simulink model "HyperscaleDataCenter"  (R2025b)
settings: Solver=VariableStepAuto  StartTime=0.0  StopTime=10  FixedStep=5e-5  RelTol=1e-4
PostLoadFcn:
  | HyperscaleDataCenterParam
values from neighbouring files (symbols this model uses):
  baseVoltageDC = 800    [DataCenterBBUParam.m]    (also in HyperscaleDataCenterParam.m; UPSBESSParam.m)
  bess_Ki = bess.controller.Ki    [SSTBESSParam.m]
  bess_Kp = bess.controller.Kp    [SSTBESSParam.m]
  droopGain = 0.02    [HyperscaleDataCenterParam.m]    (also in SSTBESSParam.m; UPSBESSParam.m)
  peakShavingPowerLimit = 800e3    (= 800000)    [HyperscaleDataCenterParam.m]
  powerTau = 0.005    [HyperscaleDataCenterParam.m]
  Prated_batt = 40e3    (= 40000)    [HyperscaleDataCenterParam.m]
  tauPS = 0.1    [HyperscaleDataCenterParam.m]
  Ts = 50e-6    (= 5e-05)    [BBUParam.m]    (also in DataCenterBBUParam.m; HyperscaleDataCenterParam.m)
  Ts_PS = 1e-3    (= 0.001)    [HyperscaleDataCenterParam.m]
undefined symbols (not defined in the file or in its folder): bbu, DiscIntNeverNeededParam, dspblkCoreblockFVToolHelper, ee_sli_rtmsupport, gcbh, grid, rack, sst, ups
libraries: fl_lib x80, nesl_utility x42, datacenter_lib x20, ee_lib x17, simulink x10, eeGeneralControl x9, slpidlib x6, microgridRenewables_lib x4, eeTransforms x4, batteryecm_lib x3, eeSinusoidalMeasurementV2 x2, simulink_extras x1
(part 2 of 5)

== system HyperscaleDataCenter/Server Load/Racks ==
  Fault Flag : Step  Time=100  SampleTime=0
  Inference Load Profile : simulink/Sources/Repeating Sequence Stair  OutValues=[0.45 0.45 0.45 0.45 0.45 0.45 0.45 0.45 0.45 0.45 0.45 0.45 0.45 0.45 0.45 0.45 0.45 0.45 0.45 0.45 0.45 0.45 0.45 0.45 0.45 0.45 0.45 0.45 0.45 0.45 0.45 0.45 0.45 0.45 0.45 0.45 0.45 0.45 0.45 0.45 0.45 0.45 0.45 0.45 0.45 0.45 0.45 0.45 0.45 0.45 0.45 0.45 0.45 0.45 0.45 0.45 0.45 0.45 0.45 0.45 0.45 0.45 0.45 0.45 0.45 0.45 0.45 0.45 0.45 0.45 0.45 0.45 0.45 0.45 0.45 0.45 0.45 0.45 0.45 0.45 0.45 0.45 0.45 0.45 0.45 0.45 0.45 0.45 0.45 0.45 0.45 0.45 0.45 0.45 0.45 0.45 0.45 0.45 0.45 0.45 0.45 0.45 0.45 0.45 0.45 0.45 0.45 0.45 0.45 0.45 0.45 0.45 0.45 0.45 0.45 0.45 0.45 0.45 0.45 0.45 0.45 0.45 0.45 0.45 0.45 0.45 0.45 0.45 0.45 0.45 0.45 0.45 0.45 0.45 0.45 0.45 0.45 0.45 0.45 0.45 0.45 0.45 0.45 0.45 0.45 0.45 0.45 0.45 0.45 0.45 0.45 0.45 0.45 0.45 0.45 0.45 0.45 0.45 0.45 0.45 0.45 0.45 0.45 0.45 0.45 0.45 0.45 0.45 0.45 0.45 0.45 0.45 0.45 0.45 0.45 0.45 0.45 0.45 0.45 0.45 0.45 0.45 0.45 0.45 0.45 0.45 0.45 0.45 0.45 0.45 0.45 0.45 0.45 0.45 0.45 0.45 0.45 0.45 0.45 0.45 0.09792 0.8812 0.4279 0.4233 0.3951 0.4417 0.4922 0.06292 0.07732 0.07716 0.08177 0.1021 0.07545 0.07538 0.0924 0.07838 0.07719 0.07756 0.07213 0.06917 0.07997 0.07917 0.09005 0.08372 0.8883 0.395 0.4378 0.3804 0.4688 0.4112 0.435 0.4169 0.4791 0.4658 0.06822 0.08707 0.06749 0.09019 0.07126 0.0691 0.0677 0.07873 0.0822 0.06972 0.09072 0.08156 0.8746 0.8709 0.4262 0.4091 0.4048 0.4395 0.4748 0.4245 0.4055 0.4479 0.429 0.3665 0.4045 0.4714 0.4592 0.412 0.4376 0.4419 0.471 0.4189 0.07003 0.04838 0.895 0.8492 0.3764 0.3779 0.4436 0.4654 0.4773 0.4169 0.4407 0.4152 0.425 0.4544 0.3988 0.403 0.4129 0.4294 0.4127 0.4608 0.448 0.5082 0.488 0.07604 0.07374 0.8828 0.8487 0.8895 0.8686 0.4234 0.4136 0.4116 0.4926 0.4523 0.4112 0.4573 0.4259 0.4585 0.4447 0.4258 0.3953 0.4105 0.4388 0.4452 0.4246 0.4057 0.4629 0.461 0.4449 0.4118 0.4226 0.3916 0.4792 0.4054 0.4544 0.4422 0.4546 0.4636 0.4855 0.4428 0.4343 0.4361 0.4804 0.496 0.4654 0.08359 0.05836 0.9365 0.8733 0.8654 0.8816 0.3909 0.3729 0.4338 0.408 0.4353 0.4173 0.4143 0.4129 0.4105 0.4518 0.4138 0.4419 0.4321 0.4582 0.4547 0.4547 0.422 0.4017 0.4296 0.4526 0.3913 0.4435 0.4495 0.4317 0.4677 0.4235 0.4225 0.4667 0.4516 0.4693 0.4495 0.4467 0.4675 0.4545 0.4623 0.4515 0.06221 0.04899 0.9312 0.8749 0.8663 0.8873 0.926 0.905 0.9178 0.4357 0.4379 0.4777 0.3905 0.4219 0.397 0.4112 0.4424 0.5089 0.4003 0.4322 0.4532 0.4096 0.4489 0.42 0.4478 0.4644 0.4798 0.4303 0.4447 0.4595 0.4207 0.4654 0.3944 0.4434 0.4156 0.41 0.3876 0.4556 0.4292 0.4569 0.4059 0.4228 0.4467 0.471 0.4269 0.4556 0.4737 0.4611 0.4292 0.4135 0.5131 0.4519 0.5096 0.4613 0.4618 0.4503 0.4521 0.465 0.4763 0.4887 0.4663 0.452 0.4517 0.4822 0.4565 0.4513 0.07011 0.06193 0.8485 0.8057 0.8966 0.8706 0.8889 0.8317 0.9382 0.8992 0.8382 0.8641 0.9356 0.9258 0.8751 0.9035 0.3864 0.4364 0.4714 0.4297 0.4344 0.4233 0.4155 0.4023 0.4171 0.3797 0.4569 0.41 0.3875 0.4516 0.458 0.465 0.4682 0.4113 0.422 0.4504 0.4696 0.3887 0.4557 0.4087 0.4055 0.435 0.4462 0.4446 0.4058 0.4619 0.4235 0.4096 0.4491 0.4915 0.4487 0.459 0.4611 0.4459 0.4174 0.4369 0.4407 0.4201 0.4502 0.4439 0.3833 0.4343 0.4686 0.3734 0.4581 0.447 0.4466 0.4605 0.4764 0.4359 0.4648 0.4588 0.4284 0.482 0.4881 0.4619 0.4698 0.4712 0.468 0.4737 0.4825 0.4637 0.4685 0.4701 0.4169 0.5148 0.487 0.4029 0.08186 0.07302 0.9172 0.454 0.4338 0.4223 0.4524 0.0829 0.09584 0.08212 0.07362 0.0809 0.08177 0.08467 0.07087 0.08213 0.08117 0.1012 0.07572 0.08253 0.09758 0.06311 0.09566 0.8076 0.4108 0.4467 0.3881 0.4411 0.4352 0.4492 0.3972 0.5191 0.5043 0.09358 0.08902 0.06735 0.08693 0.07385 0.05875 0.07534 0.0795 0.08597 0.08079 0.07329 0.1075 0.0587 0.9195 0.8938 0.3881 0.3788 0.4343 0.4336 0.4024 0.4979 0.4252 0.4297 0.4954 0.4318 0.4639 0.4354 0.432 0.4799 0.4474 0.4941 0.4304 0.4456 0.05767 0.07131 0.9125 0.8774 0.4413 0.4065 0.4383 0.4395 0.4492 0.4592 0.4394 0.45 0.417 0.3811 0.5062 0.4515 0.4701 0.4504 0.4205 0.4655 0.4519 0.4443 0.07985 0.08406 0.8564 0.9054 0.8433 0.418 0.3852 0.3823 0.4163 0.4218 ...(+2623 chars)]  tsamp=0.01  OutMin=[]  OutMax=[]  OutDataTypeStr=double  OutputDataTypeScalingMode=double  OutDataType=fixdt(0,8)  ConRadixGroup=Best Precision: Vector-wise  OutScaling=2^-12
  Inference Rack : Subsystem
  PS Step : fl_lib/Physical Signals/Sources/PS Step  step_time=100 s  initial_value=1  final_value=0
  SPST Switch : ee_lib/Switches & Breakers/SPST Switch  R_closed=0.001 Ohm  G_open=1e-6 S  Threshold=0.5 V  Width=0 V  model_dynamics=0  t_on=1e-3 s  t_off=1e-3 s  initial_vT=0 V
      settings: InternalSimscapePortConfiguration="{\"Bottom\":[],\"Left\":[{\"id\":\"vT\",\"label\":\"vT\",\"type\":\"input\"},{\"id\":\"p\",\"label\":\"\",\"type\":\"foundation.electrical.electrical\"}],\"Right\":[{\"id\":\"n\",\"label\":\"\",\"type\":\"foundation.electrical.electrical\"}],\"Top\":[]}"
  Training Load Profile : simulink/Sources/Repeating Sequence Stair  OutValues=[0.45 0.45 0.45 0.45 0.45 0.45 0.45 0.45 0.45 0.45 0.45 0.45 0.45 0.45 0.45 0.45 0.45 0.45 0.45 0.45 0.45 0.45 0.45 0.45 0.45 0.45 0.45 0.45 0.45 0.45 0.45 0.45 0.45 0.45 0.45 0.45 0.45 0.45 0.45 0.45 0.45 0.45 0.45 0.45 0.45 0.45 0.45 0.45 0.45 0.45 0.45 0.45 0.45 0.45 0.45 0.45 0.45 0.45 0.45 0.45 0.45 0.45 0.45 0.45 0.45 0.45 0.45 0.45 0.45 0.45 0.45 0.45 0.45 0.45 0.45 0.45 0.45 0.45 0.45 0.45 0.45 0.45 0.45 0.45 0.45 0.45 0.45 0.45 0.45 0.45 0.45 0.45 0.45 0.45 0.45 0.45 0.45 0.45 0.45 0.45 0.45 0.45 0.45 0.45 0.45 0.45 0.45 0.45 0.45 0.45 0.45 0.45 0.45 0.45 0.45 0.45 0.45 0.45 0.45 0.45 0.45 0.45 0.45 0.45 0.45 0.45 0.45 0.45 0.45 0.45 0.45 0.45 0.45 0.45 0.45 0.45 0.45 0.45 0.45 0.45 0.45 0.45 0.45 0.45 0.45 0.45 0.45 0.45 0.45 0.45 0.45 0.45 0.45 0.45 0.45 0.45 0.45 0.45 0.45 0.45 0.45 0.45 0.45 0.45 0.45 0.45 0.45 0.45 0.45 0.45 0.45 0.45 0.45 0.45 0.45 0.45 0.45 0.45 0.45 0.45 0.45 0.45 0.45 0.45 0.45 0.45 0.45 0.45 0.45 0.45 0.45 0.45 0.45 0.45 0.45 0.45 0.45 0.45 0.45 0.45 0.04462 0.05867 0.05976 0.05337 0.8301 0.8395 0.8241 0.8683 0.8535 0.8651 0.8382 0.8869 0.8863 0.8475 0.8278 0.8364 0.8503 0.8488 0.8368 0.8561 0.8418 0.8244 0.8443 0.8487 0.87 0.834 0.8518 0.8555 0.8073 0.8581 0.8308 0.8435 0.8996 0.8808 0.9365 0.9168 0.9028 0.928 0.9155 0.8937 0.9196 0.9024 0.9422 0.9107 0.9333 0.9094 0.9208 0.9231 0.9136 0.9629 0.936 0.9439 0.962 0.9278 0.9409 0.8926 0.9008 0.8666 0.9039 0.911 0.9053 0.9423 0.9029 0.9048 0.922 0.903 0.9312 0.9131 0.9474 0.9348 0.1393 0.1621 0.1647 0.1641 0.1161 0.1423 0.1202 0.1752 0.1554 0.1462 0.03853 0.04299 0.04355 0.05782 0.8563 0.8755 0.8485 0.8039 0.8697 0.8705 0.8526 0.862 0.8499 0.8518 0.8477 0.8228 0.8343 0.8033 0.8582 0.8377 0.8507 0.8641 0.8327 0.8442 0.8603 0.82 0.8209 0.834 0.8171 0.8803 0.8646 0.8542 0.8717 0.8626 0.9025 0.9584 0.9219 0.9301 0.9405 0.9014 0.9022 0.9003 0.9194 0.9374 0.9017 0.9207 0.915 0.8988 0.9028 0.9129 0.9366 0.9126 0.9212 0.9312 0.9165 0.941 0.9403 0.901 0.9198 0.913 0.8863 0.899 0.9338 0.9201 0.9109 0.9087 0.9491 0.9004 0.8974 0.9194 0.1738 0.1368 0.1536 0.1603 0.1415 0.1648 0.1441 0.1628 0.1555 0.1524 0.03233 0.05598 0.04442 0.03802 0.8071 0.8545 0.8574 0.8124 0.8511 0.836 0.8543 0.8144 0.8604 0.8429 0.8897 0.823 0.8373 0.8342 0.8774 0.8788 0.8398 0.856 0.8909 0.8535 0.8513 0.8096 0.8015 0.876 0.8889 0.8552 0.8426 0.8384 0.8708 0.8871 0.9413 0.9475 0.9331 0.875 0.8913 0.9496 0.9272 0.8941 0.8764 0.9402 0.897 0.9037 0.923 0.9311 0.9422 0.9095 0.9235 0.9039 0.9133 0.9329 0.9321 0.9474 0.9276 0.9244 0.8947 0.9106 0.9096 0.9026 0.9796 0.9135 0.9597 0.9275 0.9351 0.9202 0.9257 0.9193 0.1403 0.1602 0.139 0.1204 0.1525 0.1146 0.1697 0.1657 0.1804 0.1421 0.02264 0.06067 0.04766 0.06556 0.9084 0.8597 0.8401 0.8455 0.8659 0.8389 0.8325 0.8531 0.8901 0.871 0.8519 0.8336 0.8585 0.8754 0.834 0.8509 0.8686 0.8723 0.8567 0.8657 0.8408 0.8402 0.8673 0.8638 0.8755 0.8616 0.8501 0.8501 0.8618 0.854 0.931 0.9269 0.9581 0.9168 0.9116 0.8967 0.9258 0.8969 0.9188 0.9255 0.9006 0.9285 0.8993 0.9102 0.9354 0.911 0.9015 0.922 0.9323 0.8861 0.9272 0.8821 0.9023 0.9217 0.9231 0.9247 0.9276 0.9776 0.9213 0.9161 0.9361 0.907 0.9151 0.9014 0.9016 0.933 0.1643 0.1611 0.1483 0.1246 0.1351 0.1419 0.1511 0.1562 0.163 0.1382 0.06428 0.05871 0.05155 0.05442 0.8481 0.8333 0.8448 0.8584 0.8254 0.8387 0.8364 0.8278 0.8948 0.8577 0.8496 0.8168 0.8493 0.8486 0.8307 0.8452 0.8476 0.8629 0.8632 0.8297 0.8481 0.8635 0.8502 0.873 0.862 0.8265 0.8026 0.8657 0.8049 0.8561 0.9582 0.9256 0.9125 0.9248 0.9163 0.9241 0.9512 0.9099 0.9535 0.9364 0.906 0.9023 0.8988 0.9098 0.9292 0.8887 0.9103 0.9459 0.8959 0.9341 0.9067 0.8909 0.9301 0.934 0.9283 0.9331 0.9562 0.9058 0.9018 0.9366 0.9405 0.959 0.9171 0.9144 0.9386 0.9049 0.04418 0.03775 0.02733 0.04007 0.03547 0.01946 0.04286 0.03016 0.0388 0.02572 0.05602 0.04867 0.02169 0.06863 0.829 0.8294 0.8837 0.8772 0.8545 0.8538 0.8485 0.8357 0.8388 0.8571 0.8782 0.8747 0.8593 0.8062 0.8493 0.7853 0.8512 0.8453 0.8751 0.8385 0.8044 0.8229 0.8738 0.8612 0.8137 ...(+2573 chars)]  tsamp=0.01  OutMin=[]  OutMax=[]  OutDataTypeStr=double  OutputDataTypeScalingMode=double  OutDataType=fixdt(0,8)  ConRadixGroup=Best Precision: Vector-wise  OutScaling=2^-12
  Training Rack : Subsystem
  + : PMIOPort  Side=Left
  - : PMIOPort  Port=2  Side=Left
  wires:
  Training Load Profile/1 -> Training Rack/1(U_in)
  Inference Load Profile/1 -> Inference Rack/1(U_in)
  Fault Flag/1 -> Inference Rack/2(FaultFlag), Training Rack/2(FaultFlag)
  connections:
  SPST Switch/RConn1 -- Training Rack/LConn1
  PS Step/RConn1 -- SPST Switch/LConn1
  +/RConn1 -- SPST Switch/LConn2 -- Inference Rack/LConn1
  Training Rack/LConn2 -- -/RConn1 -- Inference Rack/LConn2

== system HyperscaleDataCenter/Solid State Transformer/Converters ==
  note: DAB Phase shift signal
  note: Reference signal for H-Bridge
  mabc : Inport
  phi : Inport  Port=2
  Add : Sum  Inputs=+++
  Add1 : Sum  Inputs=+++
  Bus Creator : BusCreator  Inputs=5
  Demux : Demux  Outputs=3
  Demux1 : Demux  Outputs=3
  Electrical Reference1 : fl_lib/Electrical/Electrical Elements/Electrical Reference
  Gain_1_1 : Gain  Gain=1/3
  Gain_1_3 : Gain  Gain=1/3
  Phase Splitter : ee_lib/Connectors & References/Phase Splitter
  Subsystem1 : Subsystem
  Subsystem2 : Subsystem
  Subsystem3 : Subsystem
  ABC2 : PMIOPort  Side=Left
  + : PMIOPort  Port=2  Side=Right
  - : PMIOPort  Port=3  Side=Right
  Vdc : Outport
  VdcMeas : Outport  Port=2
  wires:
  Subsystem1/1(Out1) -> Bus Creator/1, Add/1  "AVdc"
  Subsystem2/1(Out1) -> Add/2, Bus Creator/2  "BAVdc"
  Subsystem3/1(Out1) -> Bus Creator/3, Add/3  "CVdc"
  Add/1 -> Gain_1_3/1
  Gain_1_3/1 -> VdcMeas/1, Bus Creator/4  "AvGVdc"
  Bus Creator/1 -> Vdc/1
  phi/1 -> Demux1/1
  Subsystem2/2(V_out_pu) -> Add1/2
  Subsystem1/2(V_out_pu) -> Add1/1
  Subsystem3/2(V_out_pu) -> Add1/3
  Add1/1 -> Gain_1_1/1
  Gain_1_1/1 -> Bus Creator/5  "PUVdc"
  Demux1/1 -> Subsystem1/1(PhA)
  Demux1/2 -> Subsystem2/1(PhB)
  Demux1/3 -> Subsystem3/1(PhC)
  mabc/1 -> Demux/1
  Demux/1 -> Subsystem1/2(ma)
  Demux/2 -> Subsystem2/2(mb)
  Demux/3 -> Subsystem3/2(mc)
  connections:
  Subsystem1/LConn2 -- Subsystem2/LConn2 -- Subsystem3/LConn2 -- Electrical Reference1/LConn1
  Subsystem3/LConn1 -- Phase Splitter/RConn3
  Subsystem1/LConn1 -- Phase Splitter/RConn1
  Subsystem1/RConn2 -- Subsystem3/RConn2 -- -/RConn1 -- Subsystem2/RConn2
  Subsystem2/LConn1 -- Phase Splitter/RConn2
  Subsystem1/RConn1 -- Subsystem3/RConn1 -- Subsystem2/RConn1 -- +/RConn1
  Phase Splitter/LConn1 -- ABC2/RConn1

== system HyperscaleDataCenter/Solid State Transformer/DAB Controller ==
  Vdc : Inport
  Vac : Inport  Port=2
  AND_gate : Logic  AllPortsSameDT=off  OutDataTypeStr=boolean
  AND_reset : Logic  AllPortsSameDT=off  OutDataTypeStr=boolean
  Add : Sum
  Add1 : Sum
  Add2 : Sum
  Bus Selector : BusSelector  OutputSignals=AVdc,BAVdc,CVdc,AvGVdc,PUVdc
  Bus Selector1 : BusSelector  OutputSignals=pllVmag [pu],reset
  Constant : Constant  Value=0
  DAB Balancing : Subsystem
  Error : Sum  Inputs=+-
  Mux : Mux  Inputs=3
  Mux1 : Mux  Inputs=3
  PI_central : slpidlib/PID Controller  Controller=PI  Form=Parallel  TimeDomain=Discrete-time  UseExternalTs=off  SampleTime=sst.dab.sampleTime  IntegratorMethod=Forward Euler  FilterMethod=Forward Euler  ControllerParametersSource=internal  P=sst.dab.kp  I=sst.dab.ki  UseKiTs=off  D=0  UseExternalDerivativeSource=off  N=100  UseFilter=on  TunerSelectOption=Transfer Function Based (PID Tuner App)  InitialConditionSource=internal  InitialConditionForIntegrator=0  InitialConditionForFilter=0  DifferentiatorICPrevScaledInput=0  ExternalReset=falling  TrackingMode=off  Kt=1  LimitOutput=on  SatLimitsSource=internal  UpperSaturationLimit=sst.dab.upperLimit  LowerSaturationLimit=sst.dab.lowerLimit  LinearizeAsGain=off  AntiWindupMode=none  Kb=1  LimitIntegrator=off  UpperIntegratorSaturationLimit=inf  LowerIntegratorSaturationLimit=-inf  POutMin=[]  POutMax=[]  IOutMin=[]  IOutMax=[]  DOutMin=[]  DOutMax=[]  NOutMin=[]  NOutMax=[]  SumOutMin=[]  SumOutMax=[]  SaturationOutMin=[]  SaturationOutMax=[]  PParamMin=[]  PParamMax=[]  IParamMin=[]  IParamMax=[]  DParamMin=[]  DParamMax=[]  NParamMin=[]  NParamMax=[]  KbParamMin=[]  KbParamMax=[]  KtParamMin=[]  KtParamMax=[]  KbOutMin=[]  KbOutMax=[]  KtOutMin=[]  KtOutMax=[]  IntegratorOutMin=[]  IntegratorOutMax=[]  FilterOutMin=[]  FilterOutMax=[]  SumI1OutMin=[]  SumI1OutMax=[]  SumI2OutMin=[]  SumI2OutMax=[]  SumI3OutMin=[]  SumI3OutMax=[]  SumI4OutMin=[]  SumI4OutMax=[]  SumDOutMin=[]  SumDOutMax=[]  DifferentiatorOutMin=[]  DifferentiatorOutMax=[]  FilterDiffOutCoefMin=[]  FilterDiffOutCoefMax=[]  ReciprocalOutMin=[]  ReciprocalOutMax=[]  SumDenOutMin=[]  SumDenOutMax=[]  SumNumOutMin=[]  SumNumOutMax=[]  DivideOutMin=[]  DivideOutMax=[]  UdiffTsProdOutMin=[]  UdiffTsProdOutMax=[]  NTsProdOutMin=[]  NTsProdOutMax=[]  UintegralTsProdOutMin=[]  UintegralTsProdOutMax=[]  UngainTsProdOutMin=[]  UngainTsProdOutMax=[]  ClampingZeroOutDataTypeStr=Inherit: Inherit via back propagation  ClampingZeroOutMin=[]  ClampingZeroOutMax=[]  FilterDenConstantOutDataTypeStr=Inherit: Inherit via back propagation  FilterDenConstantOutMin=[]  FilterDenConstantOutMax=[]  PCopyOutDataTypeStr=Inherit: Inherit via back propagation  PCopyOutMin=[]  PCopyOutMax=[]  NCopyOutDataTypeStr=Inherit: Inherit via back propagation  NCopyOutMin=[]  NCopyOutMax=[]  IntegratorContinuousStateAttributes=''  IntegratorStateMustResolveToSignalObject=off  IntegratorRTWStateStorageClass=Auto  FilterContinuousStateAttributes=''  FilterStateMustResolveToSignalObject=off  FilterRTWStateStorageClass=Auto  ParallelPVariant=InternalParameters  IdealPVariant=Disabled  IVariant=InternalParameters  DVariant=Disabled  IntegratorVariant=Discrete  SatVariant=Enabled  AWVariant=Passthrough  PCopyVariant=Disabled  TRVariant=Disabled  FdbkBlocksVariant=Forward  IdealPFdbkVariant=Disabled  SatFdbkVariant=Disabled  DerivativeFilterVariant=Disabled  NVariant=Disabled  NCopyVariant=Disabled_SignalSpec  FilterICVariant=Disabled  IntegratorICVariant=InternalICs  ExternalResetVariant=ExternalReset  TRSumVariant=Passthrough  SumFdbkVariant=Disabled  SumVariant=Sum_PI  TsampFilterVariant=InternalTs  TsampNgainVariant=Passthrough  TsampIntegralVariant=Disabled_SignalSpec  ExternalSaturationOutDataTypeStr=Inherit: Same as second input  DerivativeSourceVariant=Disabled  PreIntVariant=InternalPreInt
      settings: LibrarySourceBlock=simulink/Discrete/Discrete PID Controller
  StartupDelay : Step  SampleTime=0
  Switch : Switch  Criteria=u2 > Threshold  SaturateOnIntegerOverflow=off  InputSameDT=off
  VacLowRelay : Relay  OnSwitchValue=0.48  OffSwitchValue=0.42  OnOutputValue=0  OffOutputValue=1
  Vref : Constant
  phi : Outport
  wires:
  Vref/1 -> Error/1
  Error/1 -> PI_central/1
  PI_central/1 -> Add1/1, Add2/1, Add/1
  Vdc/1 -> Bus Selector/1
  Bus Selector/1 -> DAB Balancing/1(Vdc_A)  "<AVdc>"
  Bus Selector/2 -> DAB Balancing/2(Vdc_B)  "<BAVdc>"
  Bus Selector/3 -> DAB Balancing/3(Vdc_C)  "<CVdc>"
  Bus Selector/4 -> DAB Balancing/4(Vdc_avg)  "<AvGVdc>"
  Bus Selector/5 -> Error/2  "<PUVdc>"
  DAB Balancing/1(delta_d_A) -> Add/2  "delta_d_A"
  DAB Balancing/2(delta_d_B) -> Add1/2  "delta_d_B"
  DAB Balancing/3(delta_d_C) -> Add2/2  "delta_d_C"
  Add/1 -> Mux/1
  Add2/1 -> Mux/3
  Add1/1 -> Mux/2
  Mux/1 -> Switch/3
  Vac/1 -> Bus Selector1/1
  Bus Selector1/1 -> VacLowRelay/1  "<pllVmag [pu]>"
  Switch/1 -> phi/1
  Constant/1 -> Mux1/3, Mux1/2, Mux1/1
  Mux1/1 -> Switch/1
  StartupDelay/1 -> AND_gate/2, AND_reset/2
  AND_gate/1 -> Switch/2
  Bus Selector1/2 -> AND_reset/1  "<reset>"
  AND_reset/1 -> PI_central/2
  VacLowRelay/1 -> AND_gate/1

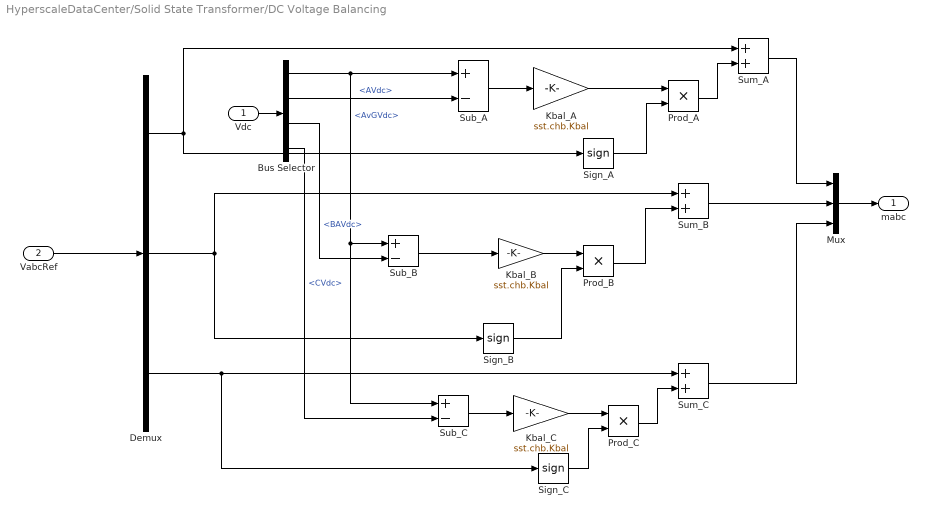
== system HyperscaleDataCenter/Solid State Transformer/DC Voltage Balancing ==
  Vdc : Inport
  VabcRef : Inport  Port=2
  Bus Selector : BusSelector  OutputSignals=AvGVdc,AVdc,BAVdc,CVdc
  Demux : Demux  Outputs=3
  Kbal_A : Gain  Gain=sst.chb.Kbal
  Kbal_B : Gain  Gain=sst.chb.Kbal
  Kbal_C : Gain  Gain=sst.chb.Kbal
  Mux : Mux  Inputs=3
  Prod_A : Product
  Prod_B : Product
  Prod_C : Product
  Sign_A : Signum
  Sign_B : Signum
  Sign_C : Signum
  Sub_A : Sum  Inputs=+-
  Sub_B : Sum  Inputs=+-
  Sub_C : Sum  Inputs=+-
  Sum_A : Sum
  Sum_B : Sum
  Sum_C : Sum
  mabc : Outport
  wires:
  Sub_B/1 -> Kbal_B/1
  Prod_B/1 -> Sum_B/2
  Sub_A/1 -> Kbal_A/1
  Sub_C/1 -> Kbal_C/1
  Kbal_A/1 -> Prod_A/1
  Sign_A/1 -> Prod_A/2
  Kbal_C/1 -> Prod_C/1
  Sign_C/1 -> Prod_C/2
  Kbal_B/1 -> Prod_B/1
  Sign_B/1 -> Prod_B/2
  Prod_A/1 -> Sum_A/2
  Prod_C/1 -> Sum_C/2
  Bus Selector/1 -> Sub_C/1, Sub_B/1, Sub_A/1  "<AvGVdc>"
  VabcRef/1 -> Demux/1
  Demux/1 -> Sum_A/1, Sign_A/1
  Demux/2 -> Sum_B/1, Sign_B/1
  Demux/3 -> Sign_C/1, Sum_C/1
  Sum_B/1 -> Mux/2
  Sum_A/1 -> Mux/1
  Sum_C/1 -> Mux/3
  Mux/1 -> mabc/1
  Vdc/1 -> Bus Selector/1
  Bus Selector/2 -> Sub_A/2  "<AVdc>"
  Bus Selector/3 -> Sub_B/2  "<BAVdc>"
  Bus Selector/4 -> Sub_C/2  "<CVdc>"

== system HyperscaleDataCenter/Solid State Transformer/Filter & AC measurements ==
  Current : Subsystem
  Current and Voltage Sensor (Three-Phase) : ee_lib/Sensors & Transducers/Current and Voltage Sensor (Three-Phase)  vMeasurementType=ee.enum.vmeasurement.lg  outputUnit=ee.enum.unit.pu  SRated=20e6 A*V  VRated=13800 V  I_specify=off  I_priority=None  I=[0, 0, 0] A  I_nominal_specify=off  I_nominal_value=1  I_nominal_unit=A  V_specify=off  V_priority=None  V=[0, 0, 0] V  V_nominal_specify=off  V_nominal_value=1  V_nominal_unit=V
      settings: InternalSimscapePortConfiguration="{\"Bottom\":[],\"Left\":[{\"id\":\"N1\",\"label\":\"~1\",\"type\":\"foundation.electrical.three_phase\"}],\"Right\":[{\"id\":\"V_output\",\"label\":\"V\",\"type\":\"output\"},{\"id\":\"I_output\",\"label\":\"I\",\"type\":\"output\"},{\"id\":\"N2\",\"label\":\"~2\",\"type\":\"foundation.electrical.three_phase\"}],\"Top\":[]}"
  Gain : Gain  Gain=1/(5e6)
  Gain1 : Gain  Gain=1/(5e6)
  Low-Pass Filter (Discrete or Continuous)1 : eeGeneralControl/Low-Pass Filter (Discrete or Continuous)  K=1  T=10e-3  B=inf  A=-inf  init_option=Inherited from block input  x0=0  Ts=-1
  Low-Pass Filter (Discrete or Continuous)2 : eeGeneralControl/Low-Pass Filter (Discrete or Continuous)  K=1  T=10e-3  B=inf  A=-inf  init_option=Inherited from block input  x0=0  Ts=-1
  PLL : Subsystem  Commented=on
      settings: PortSchema="{\"entries\":[{\"content\":{\"sides\":[{\"content\":{\"connectorIds\":[\"Out1\",\"Out2\",\"Out3\"]},\"type\":\"ConnectorPlacement.EquallySpacedRectSide\",\"uuid\":\"76485780-20fe-4fcf-8224-69648da6ed2a\"},{\"content\":{\"connectorIds\":[\"In1\",\"In2\"],\"side\":\"RIGHT\"},\"type\":\"ConnectorPlacement.EquallySpacedRectSide\",\"uuid\":\"f19a6390-e634-42c7-8d46-4cd80cbab182\"},{\"content\":{\"side\":\"TOP\"},\"type\":\"ConnectorPlacement.EquallySpacedRectSide\",\"uuid\":\"87682f72-1844-428e-be70-ad7ca3191ee3\"}]},\"type\":\"ConnectorPlacement.EquallySpacedConnector\",\"uuid\":\"f2136b07-48ec-402b-adb3-18c0bac2157c\"}],\"packageUris\":[\"http://schema.mathworks.com/mf0/Connector/R2020b\"],\"version\":\"1.0\"}"
  PS-Simulink Converter : nesl_utility/PS-Simulink Converter  PhysicalDomain=network_engine_domain  SubClassName=ps_output  LeftPortType=input  RightPortType=output  PseudoPeriodic=off  Frequencies=[]  VectorFormat=1-D array  Unit=inherit  AffineConversion=off
  PS-Simulink Converter1 : nesl_utility/PS-Simulink Converter  PhysicalDomain=network_engine_domain  SubClassName=ps_output  LeftPortType=input  RightPortType=output  PseudoPeriodic=off  Frequencies=[]  VectorFormat=1-D array  Unit=inherit  AffineConversion=off
  PS-Simulink Converter2 : nesl_utility/PS-Simulink Converter  PhysicalDomain=network_engine_domain  SubClassName=ps_output  LeftPortType=input  RightPortType=output  PseudoPeriodic=off  Frequencies=[]  VectorFormat=inherit  Unit=inherit  AffineConversion=off
  PS-Simulink Converter3 : nesl_utility/PS-Simulink Converter  PhysicalDomain=network_engine_domain  SubClassName=ps_output  LeftPortType=input  RightPortType=output  PseudoPeriodic=off  Frequencies=[]  VectorFormat=inherit  Unit=inherit  AffineConversion=off
  Power Sensor (Three-Phase) : ee_lib/Sensors & Transducers/Power Sensor (Three-Phase)  load_type=ee.enum.passive.type_balanced.balanced  f0=60 Hz
      settings: InternalSimscapePortConfiguration="{\"Bottom\":[],\"Left\":[{\"id\":\"N1\",\"label\":\"~1\",\"type\":\"foundation.electrical.three_phase\"}],\"Right\":[{\"id\":\"N2\",\"label\":\"~2\",\"type\":\"foundation.electrical.three_phase\"}],\"Top\":[{\"id\":\"Pm\",\"label\":\"P\",\"type\":\"output\"},{\"id\":\"Qm\",\"label\":\"Q\",\"type\":\"output\"}]}"
  RL filter : ee_lib/Passive/RLC Assemblies/RLC (Three-Phase)  port_option=ee.enum.threePhasePort.composite  component_structure=ee.enum.rlc.structure.SeriesRL  R=0.1 Ohm  L=0.01 H  C=1e-6 F  R_parasitic=1e-6 Ohm  G_parasitic=1e-6 1/Ohm  IL_specify=on  IL_priority=None  IL=[0, 0, 0] A  IL_nominal_specify=off  IL_nominal_value=1  IL_nominal_unit=A  VC_specify=on  VC_priority=None  VC=[0, 0, 0] V  VC_nominal_specify=off  VC_nominal_value=1  VC_nominal_unit=V
      settings: InternalSimscapePortConfiguration="{\"Bottom\":[],\"Left\":[{\"id\":\"N1\",\"label\":\"~1\",\"type\":\"foundation.electrical.three_phase\"}],\"Right\":[{\"id\":\"N2\",\"label\":\"~2\",\"type\":\"foundation.electrical.three_phase\"}],\"Top\":[]}"
  Terminator : Terminator
  Terminator1 : Terminator
  Voltage : Subsystem
  ABC : PMIOPort  Side=Left
  ABC2 : PMIOPort  Port=2  Side=Right
  Vabc : Outport
  Iabc : Outport  Port=2
  wires:
  PS-Simulink Converter/1 -> Current/1(Isabc)
  Current/1(Iabc) -> Iabc/1, PLL/1(Iabc)
  PS-Simulink Converter1/1 -> Voltage/1(Vsabc)
  Voltage/1(Vabc) -> Vabc/1, PLL/2(V)
  PS-Simulink Converter2/1 -> Gain/1
  PS-Simulink Converter3/1 -> Gain1/1
  Gain/1 -> Low-Pass Filter (Discrete or Continuous)1/1
  Gain1/1 -> Low-Pass Filter (Discrete or Continuous)2/1
  PLL/3(mag) -> ?
  PLL/2(freq) -> ?
  Low-Pass Filter (Discrete or Continuous)1/1 -> Terminator/1
  Low-Pass Filter (Discrete or Continuous)2/1 -> Terminator1/1
  connections:
  Current and Voltage Sensor (Three-Phase)/RConn2 -- PS-Simulink Converter/LConn1
  PS-Simulink Converter1/LConn1 -- Current and Voltage Sensor (Three-Phase)/RConn1
  Current and Voltage Sensor (Three-Phase)/LConn1 -- ABC/RConn1
  Power Sensor (Three-Phase)/RConn1 -- RL filter/LConn1
  Power Sensor (Three-Phase)/LConn2 -- PS-Simulink Converter2/LConn1
  Power Sensor (Three-Phase)/LConn3 -- PS-Simulink Converter3/LConn1
  RL filter/RConn1 -- ABC2/RConn1
  Power Sensor (Three-Phase)/LConn1 -- Current and Voltage Sensor (Three-Phase)/RConn3

== system HyperscaleDataCenter/Solid State Transformer/PFC Rectifier Controller ==
  VdcRef (V) : Inport
  QRef (pu) : Inport  Port=2
  VdcSens (V) : Inport  Port=3
  VabcSens (pu) : Inport  Port=4
  IabcSens (pu) : Inport  Port=5
  Current Controller : Subsystem
  DC Voltage Controller and Current Reference : Subsystem
  PLL : Subsystem
      settings: PortSchema="{\"entries\":[{\"content\":{\"sides\":[{\"content\":{\"connectorIds\":[\"Out1\",\"Out2\",\"Out3\",\"Out4\"]},\"type\":\"ConnectorPlacement.EquallySpacedRectSide\",\"uuid\":\"76485780-20fe-4fcf-8224-69648da6ed2a\"},{\"content\":{\"connectorIds\":[\"In1\"],\"side\":\"RIGHT\"},\"type\":\"ConnectorPlacement.EquallySpacedRectSide\",\"uuid\":\"f19a6390-e634-42c7-8d46-4cd80cbab182\"},{\"content\":{\"side\":\"TOP\"},\"type\":\"ConnectorPlacement.EquallySpacedRectSide\",\"uuid\":\"87682f72-1844-428e-be70-ad7ca3191ee3\"}]},\"type\":\"ConnectorPlacement.EquallySpacedConnector\",\"uuid\":\"f2136b07-48ec-402b-adb3-18c0bac2157c\"}],\"packageUris\":[\"http://schema.mathworks.com/mf0/Connector/R2020b\"],\"version\":\"1.0\"}"
  Rate Transition : RateTransition  InitialCondition=1  OutPortSampleTime=Ts
  Reset Controller : Subsystem
  VabcRef (pu) : Outport
  Out Bus Element : Outport  Port=2  PortName=Visualization  Element=pllAngle [rad]
  Out Bus Element1 : Outport  Port=2  PortName=Visualization  Element=pllVmag [pu]
  Out Bus Element2 : Outport  Port=2  PortName=Visualization  Element=Idref [pu]
  Out Bus Element3 : Outport  Port=2  PortName=Visualization  Element=Iqref [pu]
  Out Bus Element5 : Outport  Port=2  PortName=Visualization  Element=IdCntrlError [pu]
  Out Bus Element6 : Outport  Port=2  PortName=Visualization  Element=IqCntrlError [pu]
  BusElementOut : Outport  Port=2  PortName=Visualization  Element=reset
  Flag : Outport  Port=3
  wires:
  Current Controller/3(IqCntrlError) -> Out Bus Element6/1
  Current Controller/2(IdCntrlError) -> Out Bus Element5/1
  PLL/1(theta) -> Out Bus Element/1, Current Controller/3(theta)
  Rate Transition/1 -> PLL/1(V)
  DC Voltage Controller and Current Reference/2(iqRef) -> Current Controller/2(iqRef), Out Bus Element3/1
  DC Voltage Controller and Current Reference/1(idRef) -> Out Bus Element2/1, Current Controller/1(idRef)
  IabcSens (pu)/1 -> Current Controller/6(iabc(PU))
  PLL/3(Vq) -> Current Controller/5(vq)
  VdcSens (V)/1 -> DC Voltage Controller and Current Reference/4(VdcSens)
  Current Controller/1(vabcRef) -> VabcRef (pu)/1
  PLL/4(mag) -> Current Controller/7(Vmag), Reset Controller/1(u), DC Voltage Controller and Current Reference/2(vPeak), Out Bus Element1/1
  QRef (pu)/1 -> DC Voltage Controller and Current Reference/1(qRef)
  VabcSens (pu)/1 -> Rate Transition/1
  VdcRef (V)/1 -> DC Voltage Controller and Current Reference/3(vdcRef)
  PLL/2(Vd) -> Current Controller/4(vd)
  Current Controller/4(Flag) -> Flag/1
  Reset Controller/1(Out1) -> Current Controller/8(Reset), BusElementOut/1, DC Voltage Controller and Current Reference/5(Reset)

== system HyperscaleDataCenter/Battery Energy Storage/BESS/DC-DC Converter Controller ==
  Voref : Inport
  Vo : Inport  Port=2
  Vac : Inport  Port=3
  iPeakShave : Inport  Port=4
  Flag : Inport  Port=5
  Current Reference Generator : Subsystem
  Gain : Gain  Gain=18750
  Mode Control : Subsystem
  Saturation : Saturate  UpperLimit=0  LowerLimit=-40000
  Simulink-PS Converter : nesl_utility/Simulink-PS Converter  PhysicalDomain=network_engine_domain  SubClassName=ps_input  LeftPortType=input  RightPortType=output  PseudoPeriodic=off  Frequencies=[]  NoiseDistribution=none  NoiseParameters=[]  Unit=1  AffineConversion=off  FilteringAndDerivatives=filter  SimscapeFilterOrder=1  InputFilterTimeConstant=0.001  UdotUserProvided=0
  mod : PMIOPort  Side=Right
  wires:
  Gain/1 -> Saturation/1
  Vac/1 -> Mode Control/2(Vac)
  Current Reference Generator/1(i) -> Gain/1
  Mode Control/1(DischargeFlag) -> Current Reference Generator/2(DischargeFlag)
  Saturation/1 -> Simulink-PS Converter/1
  Vo/1 -> Mode Control/1(Vdc)
  Mode Control/3(iRef) -> Current Reference Generator/4(I)
  Voref/1 -> Current Reference Generator/1(VoRef)
  iPeakShave/1 -> Current Reference Generator/6(iPeakShave)
  Mode Control/2(vOut) -> Current Reference Generator/3(Vo)
  Flag/1 -> Current Reference Generator/5(Mode)
  connections:
  mod/RConn1 -- Simulink-PS Converter/RConn1

== system HyperscaleDataCenter/HV Substation/Transformer/Detailed ==
  Two-Winding Transformer (Three-Phase) : ee_lib/Passive/Transformers/Two-Winding Transformer (Three-Phase)  SRated=100e6 A*V  FRated=grid.frequency Hz  Winding1Connection=ee.enum.windingconnection.Yg  VRated1=grid.voltage V  Winding2Connection=ee.enum.windingconnection.Yg  VRated2=13800 V  CoreType=ee.enum.coretype.threelimb  pu_Rw1=0.01  pu_Rw2=0.01  leakage_reactance_option=ee.enum.transformer_leakage.include  pu_Xl1=0.05  pu_Xl2=0.05  magnetizing_resistance_option=ee.enum.transformer_magnetizingResistance.exclude  pu_Rm=500  magnetizing_reactance_option=ee.enum.transformer_magnetizingReactance.exclude  saturation_option=ee.enum.transformer_saturation.exclude  pu_Xm=500  current_data=[0, .002, 1, 2]  magnetic_flux_data=[0, 1.2, 1.5, 1.51]  pu_X0=0.5  i1_specify=off  i1_priority=None  i1=[0, 0, 0] A  i1_nominal_specify=off  i1_nominal_value=1  i1_nominal_unit=A  i2_specify=off  i2_priority=None  i2=[0, 0, 0] A  i2_nominal_specify=off  i2_nominal_value=1  i2_nominal_unit=A  phi_specify=off  phi_priority=None  phi=[0, 0, 0]  phi_nominal_specify=off  phi_nominal_value=1  phi_nominal_unit=1  power_dissipated_specify=off  power_dissipated_priority=None  power_dissipated=0 W  power_dissipated_nominal_specify=off  power_dissipated_nominal_value=1  power_dissipated_nominal_unit=W
      settings: InternalSimscapePortConfiguration="{\"Bottom\":[],\"Left\":[{\"id\":\"N1\",\"label\":\"~1\",\"type\":\"foundation.electrical.three_phase\"}],\"Right\":[{\"id\":\"N2\",\"label\":\"~2\",\"type\":\"foundation.electrical.three_phase\"}],\"Top\":[]}"
  In : PMIOPort  Side=Left
  Out : PMIOPort  Port=2  Side=Right
  connections:
  Two-Winding Transformer (Three-Phase)/LConn1 -- In/RConn1
  Two-Winding Transformer (Three-Phase)/RConn1 -- Out/RConn1

== system HyperscaleDataCenter/HV Substation/Transformer/Simplified ==
  Electrical Reference : fl_lib/Electrical/Electrical Elements/Electrical Reference
  Electrical Reference1 : fl_lib/Electrical/Electrical Elements/Electrical Reference
  Ideal Transformer : fl_lib/Electrical/Electrical Elements/Ideal Transformer  n=windingRatio  i1_specify=off  i1_priority=None  i1=0 A  i1_nominal_specify=off  i1_nominal_value=1  i1_nominal_unit=A  v1_specify=off  v1_priority=None  v1=0 V  v1_nominal_specify=off  v1_nominal_value=1  v1_nominal_unit=V  i2_specify=off  i2_priority=None  i2=0 A  i2_nominal_specify=off  i2_nominal_value=1  i2_nominal_unit=A  v2_specify=off  v2_priority=None  v2=0 V  v2_nominal_specify=off  v2_nominal_value=1  v2_nominal_unit=V
  Ideal Transformer1 : fl_lib/Electrical/Electrical Elements/Ideal Transformer  n=windingRatio  i1_specify=off  i1_priority=None  i1=0 A  i1_nominal_specify=off  i1_nominal_value=1  i1_nominal_unit=A  v1_specify=off  v1_priority=None  v1=0 V  v1_nominal_specify=off  v1_nominal_value=1  v1_nominal_unit=V  i2_specify=off  i2_priority=None  i2=0 A  i2_nominal_specify=off  i2_nominal_value=1  i2_nominal_unit=A  v2_specify=off  v2_priority=None  v2=0 V  v2_nominal_specify=off  v2_nominal_value=1  v2_nominal_unit=V
  Ideal Transformer2 : fl_lib/Electrical/Electrical Elements/Ideal Transformer  n=windingRatio  i1_specify=off  i1_priority=None  i1=0 A  i1_nominal_specify=off  i1_nominal_value=1  i1_nominal_unit=A  v1_specify=off  v1_priority=None  v1=0 V  v1_nominal_specify=off  v1_nominal_value=1  v1_nominal_unit=V  i2_specify=off  i2_priority=None  i2=0 A  i2_nominal_specify=off  i2_nominal_value=1  i2_nominal_unit=A  v2_specify=off  v2_priority=None  v2=0 V  v2_nominal_specify=off  v2_nominal_value=1  v2_nominal_unit=V
  Phase Splitter : ee_lib/Connectors & References/Phase Splitter
  Phase Splitter1 : ee_lib/Connectors & References/Phase Splitter
  In : PMIOPort  Side=Left
  Out : PMIOPort  Port=2  Side=Right
  connections:
  Ideal Transformer/RConn2 -- Electrical Reference1/LConn1 -- Ideal Transformer1/RConn2 -- Ideal Transformer2/RConn2
  Phase Splitter/RConn3 -- Ideal Transformer2/LConn1
  Phase Splitter/RConn2 -- Ideal Transformer1/LConn1
  Phase Splitter/RConn1 -- Ideal Transformer/LConn1
  Ideal Transformer/LConn2 -- Electrical Reference/LConn1 -- Ideal Transformer1/LConn2 -- Ideal Transformer2/LConn2
  Phase Splitter/LConn1 -- In/RConn1
  Phase Splitter1/LConn1 -- Out/RConn1
  Ideal Transformer/RConn1 -- Phase Splitter1/RConn1
  Ideal Transformer2/RConn1 -- Phase Splitter1/RConn3
  Ideal Transformer1/RConn1 -- Phase Splitter1/RConn2
